simulink model "TestMassAccelerometer_NonlinearModel_Simulink2017a"  (R2017a)
settings: Solver=ode4  StartTime=0.0  StopTime=SIM_TIME  FixedStep=STEP_SIZE  RelTol=1e-3
undefined symbols (not defined in the file): A, c1, c2, f1, f2, f3, f4, f5, f6, g, m, x0
settings Model: Creator=Roberto  LastModifiedBy=roga

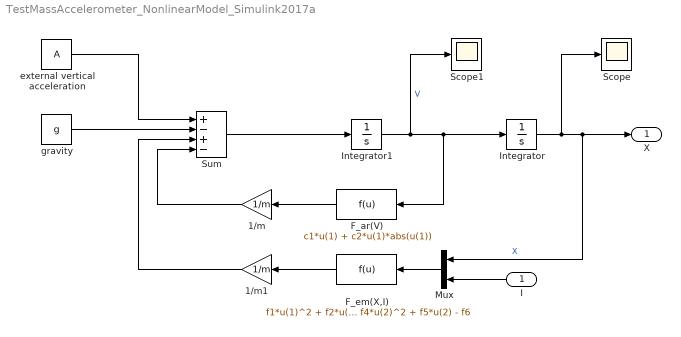
== system TestMassAccelerometer_NonlinearModel_Simulink2017a ==
  I : Inport
  1/m : Gain  Gain=1/m
  1/m1 : Gain  Gain=1/m
  F_ar(V) : Fcn  Expr=c1*u(1) + c2*u(1)*abs(u(1))
  F_em(X,I) : Fcn  Expr=f1*u(1)^2 + f2*u(1)*u(2) - f3*u(1) + f4*u(2)^2 + f5*u(2) - f6
  Integrator : Integrator  Priority=1  InitialCondition=x0(1)
  Integrator1 : Integrator  Priority=2  InitialCondition=x0(2)
  Mux : Mux  Inputs=2
  Scope : Scope
  Scope1 : Scope
  Sum : Sum  Inputs=+-+-
  external vertical acceleration : Constant  Value=A
  gravity : Constant  Value=g
  X : Outport
  wires:
  Integrator1/1 -> Scope1/1, Integrator/1, F_ar(V)/1  "V"
  Sum/1 -> Integrator1/1
  gravity/1 -> Sum/2
  external vertical acceleration/1 -> Sum/1
  Mux/1 -> F_em(X,I)/1
  Integrator/1 -> Scope/1, X/1, Mux/1  "X"
  F_em(X,I)/1 -> 1/m1/1
  F_ar(V)/1 -> 1/m/1
  1/m/1 -> Sum/4
  1/m1/1 -> Sum/3
  I/1 -> Mux/2
